simulink library "governor_lib"  (R2022b)
settings: Solver=VariableStepAuto  StartTime=0.0  StopTime=10.0  RelTol=1e-3
undefined symbols (not defined in the file): BM_STATUSES, DI_STATUSES, MI_STATUSES
settings Model: Creator=dr_pa  LastModifiedBy=LinF

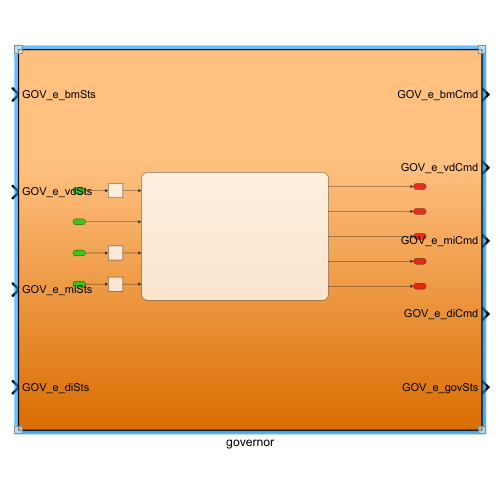
[thumbnail: Simulink's stored preview of the top-level diagram]
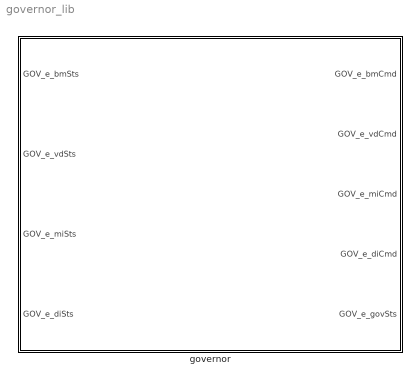
== system governor_lib ==
  governor : Subsystem

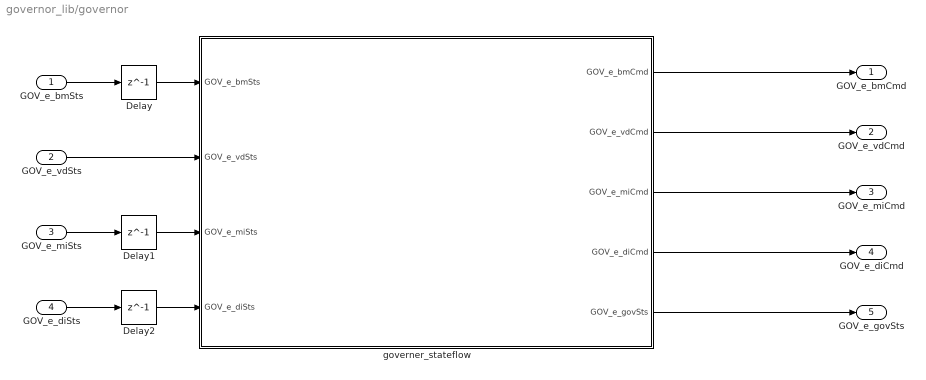
== system governor_lib/governor ==
  GOV_e_bmSts : Inport
  GOV_e_vdSts : Inport  Port=2
  GOV_e_miSts : Inport  Port=3
  GOV_e_diSts : Inport  Port=4
  Delay : Delay  DelayLength=1  InitialCondition=BM_STATUSES.BM_UNKNOWN
  Delay1 : Delay  DelayLength=1  InitialCondition=MI_STATUSES.UNKNOWN
  Delay2 : Delay  DelayLength=1  InitialCondition=DI_STATUSES.DI_UNKNOWN
  governer_stateflow : Stateflow chart  TreatAsAtomicUnit=on
  GOV_e_bmCmd : Outport
  GOV_e_vdCmd : Outport  Port=2
  GOV_e_miCmd : Outport  Port=3
  GOV_e_diCmd : Outport  Port=4
  GOV_e_govSts : Outport  Port=5
  wires:
  governer_stateflow/5(GOV_e_govSts) -> GOV_e_govSts/1
  GOV_e_bmSts/1 -> Delay/1
  GOV_e_vdSts/1 -> governer_stateflow/2(GOV_e_vdSts)
  GOV_e_diSts/1 -> Delay2/1
  governer_stateflow/1(GOV_e_bmCmd) -> GOV_e_bmCmd/1
  governer_stateflow/2(GOV_e_vdCmd) -> GOV_e_vdCmd/1
  governer_stateflow/3(GOV_e_miCmd) -> GOV_e_miCmd/1
  governer_stateflow/4(GOV_e_diCmd) -> GOV_e_diCmd/1
  GOV_e_miSts/1 -> Delay1/1
  Delay/1 -> governer_stateflow/1(GOV_e_bmSts)
  Delay1/1 -> governer_stateflow/3(GOV_e_miSts)
  Delay2/1 -> governer_stateflow/4(GOV_e_diSts)

== stateflow chart governor_lib/governor/governer_stateflow ==
  state Initialize_outputs
    en:
    GOV_e_govSts = GOV_STATUSES.GOV_INIT;
    GOV_e_diCmd = DI_CMD.DI_CMD_INIT;
    GOV_e_bmCmd = BM_CMD.BM_CMD_INIT;
    motorStartCount = 0;
  state STARTUP
    en:
    GOV_e_govSts = GOV_STATUSES.GOV_STARTUP;
    state HV_startup
      en:
      GOV_e_bmCmd = ...
      BM_CMD.HV_STARTUP;
    state ReadyToDrive
      en:
      GOV_e_diCmd = ...
      DI_CMD.HV_ON;
    state Command_motor_startup
      en:
      GOV_e_miCmd = MI_CMD.CMD_STARTUP;
      motorStartCount = motorStartCount+1;
    state Send_ReadyToDrive
      en:
      GOV_e_diCmd = DI_CMD.READY_TO_DRIVE;
    (default) -> HV_startup
    HV_startup -> ReadyToDrive : [GOV_e_bmSts == BM_STATUSES.BM_RUNNING]
    ReadyToDrive -> Command_motor_startup : [GOV_e_diSts == DI_STATUSES.READY_TO_DRIVE_REQ]
    Command_motor_startup -> Send_ReadyToDrive : [GOV_e_miSts == ...
        | MI_STATUSES.RUNNING]
  state STARTUP_ERROR
    state HV_startup_error
      en:
      GOV_e_govSts =...
      GOV_STATUSES.HV_STARTUP_ERROR;
      GOV_e_diCmd = DI_CMD.DI_SHUTDOWN;
    state Err_reset
      during:
      GOV_e_miCmd=...
      MI_CMD.ERR_RESET;
    state Motor_faulted
      en:
      % tell other motor to shutdown
      % if still running
      GOV_e_miCmd=...
      MI_CMD.CMD_SHUTDOWN;
      GOV_e_govSts =...
      GOV_STATUSES.MOTOR_STARTUP_ERROR;
    state DriverInterface_Error
      en:
      GOV_e_govSts =...
      GOV_STATUSES.GOV_DI_ERROR;
    (junction 88) -> Err_reset [order 2]
    (junction 88) -> Motor_faulted [order 1] : [motorStartCount >= 5]
  state Vehicle_shutdown
    en:
    GOV_e_govSts = GOV_STATUSES.GOV_SHUTDOWN;
    GOV_e_miCmd = MI_CMD.CMD_SHUTDOWN;
    GOV_e_diCmd = DI_CMD.DI_SHUTDOWN;
  state RUNNING_ERROR
    state HV_run_error
      en:
      GOV_e_diCmd = ...
      DI_CMD.RUN_ERROR;
      GOV_e_govSts =...
      GOV_STATUSES.HV_RUN_ERROR;
    state Motor_run_error
      en:
      GOV_e_diCmd = ...
      DI_CMD.RUN_ERROR;
      GOV_e_govSts =...
      GOV_STATUSES.MOTOR_RUN_ERROR;
  state RUNNING
    en:
    GOV_e_govSts = GOV_STATUSES.GOV_RUNNING;
  (default) -> Initialize_outputs
  HV_startup_error -> Initialize_outputs : [GOV_e_bmSts == BM_STATUSES.BM_INIT]
  Vehicle_shutdown -> Initialize_outputs : [GOV_e_bmSts == BM_STATUSES.BM_INIT]
  Initialize_outputs -> HV_startup : after(2,sec)[GOV_e_diSts == ...
      | DI_STATUSES.HV_START_REQ]
  STARTUP -> HV_startup_error [order 1] : [GOV_e_bmSts == ...
      | BM_STATUSES.HVIL_INTERRUPT]
  Err_reset -> STARTUP : [GOV_e_miSts ==...
      |  MI_STATUSES.OFF]
  STARTUP -> (junction 88) [order 3] : [GOV_e_miSts == ...
      | MI_STATUSES.MI_STS_ERROR]
  RUNNING -> Vehicle_shutdown [order 1] : [GOV_e_bmSts == BM_STATUSES.HVIL_INTERRUPT || ...
      | GOV_e_bmSts == BM_STATUSES.BM_LOW_SOC]
  STARTUP -> DriverInterface_Error [order 2] : [GOV_e_diSts ==...
      | DI_STATUSES.DI_ERROR]
  Send_ReadyToDrive -> RUNNING : [GOV_e_diSts == ...
      | DI_STATUSES.DI_RUNNING]
  RUNNING -> HV_run_error [order 2] : [GOV_e_bmSts == ...
      | BM_STATUSES.ERR_RUNNING]
  RUNNING -> Motor_run_error [order 3] : [GOV_e_miSts == ...
      | MI_STATUSES.MI_STS_ERROR]
  data: GOV_e_bmSts input; GOV_e_vdSts input; GOV_e_miSts input; GOV_e_diSts input; GOV_e_bmCmd output size=1; GOV_e_vdCmd output uint8 size=1; GOV_e_miCmd output Enum: MI_CMD size=1; GOV_e_diCmd output Enum: DI_CMD size=1; motorStartCount local uint16; GOV_e_govSts output
